simulink library "SV_pattern_generator_with_global_TRGO"  (R2025b)
settings: Solver=VariableStepAuto  StartTime=0.0  StopTime=10.0  RelTol=1e-3
undefined symbols (not defined in the file): fPWM_DAB, tc
libraries: single_phase_pwm_modulator x1
settings Model: Creator=dbagn  LastModifiedBy=dbagn

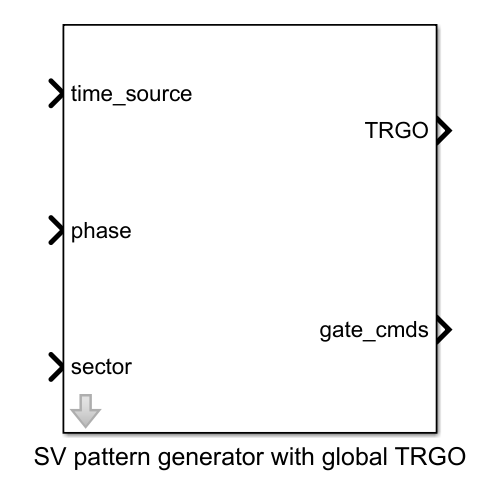
[thumbnail: Simulink's stored preview of the top-level diagram]
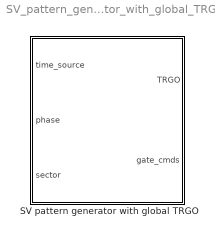
== system SV_pattern_generator_with_global_TRGO ==
  SV pattern generator with global TRGO : Subsystem  mask{f=fPWM_DAB, m_up=0.98, m_low=0.02, dead_time=0, pos_cmd_gate=15, neg_cmd_gate=-10, tc=tc}
      mask prompts: f "Frequency (Hz)"; m_up "Max Input Modulation Value"; m_low "Min Input Modulation Value"; dead_time "Dead Time (s)"; pos_cmd_gate "Positive Gate Voltage (V)"; neg_cmd_gate "Negative Gate Voltage (V)"; tc "Sampling time (s)"

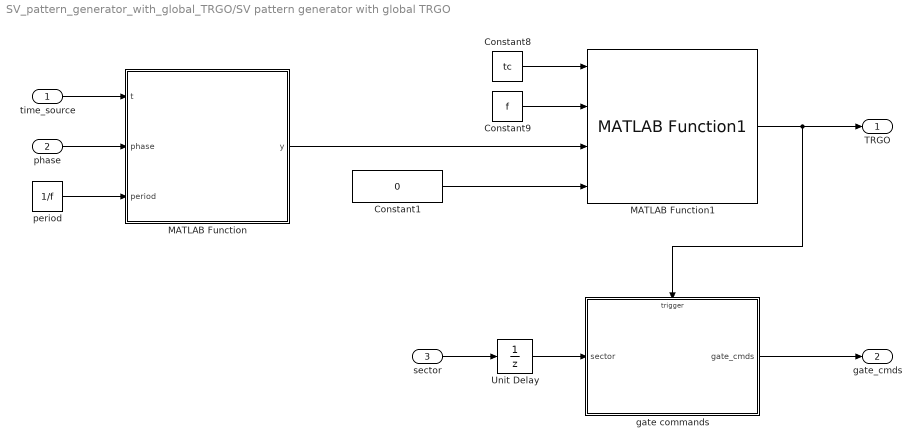
== system SV_pattern_generator_with_global_TRGO/SV pattern generator with global TRGO ==
  time_source : Inport
  phase : Inport  Port=2
  sector : Inport  Port=3
  Constant1 : Constant  Value=0
  Constant8 : Constant  Value=tc
  Constant9 : Constant  Value=f
  MATLAB Function : MATLAB Function  TreatAsAtomicUnit=on  SystemSampleTime=tc
  MATLAB Function1 : single_phase_pwm_modulator/Single phase two level PWM generator with global TRGO/MATLAB Function1  SystemSampleTime=tc  VariantActivationTime=update diagram  EmptyChoice=off  PassThrough=off  PassThroughVariantControl=(default)  EmptyChoiceVariantControl=(default)  AllowFlexibleInterface=on  Latency=0  AutoFrameSizeCalculation=off
  Unit Delay : UnitDelay  SampleTime=tc  HasFrameUpgradeWarning=on
  gate commands : Subsystem
  period : Constant  Value=1/f
  TRGO : Outport
  gate_cmds : Outport  Port=2
  wires:
  Constant1/1 -> MATLAB Function1/4
  time_source/1 -> MATLAB Function/1(t)
  gate commands/1(gate_cmds) -> gate_cmds/1
  sector/1 -> Unit Delay/1
  Constant9/1 -> MATLAB Function1/2
  Constant8/1 -> MATLAB Function1/1
  MATLAB Function/1(y) -> MATLAB Function1/3
  phase/1 -> MATLAB Function/2(phase)
  period/1 -> MATLAB Function/3(period)
  MATLAB Function1/1 -> gate commands/Trigger, TRGO/1
  Unit Delay/1 -> gate commands/1(sector)

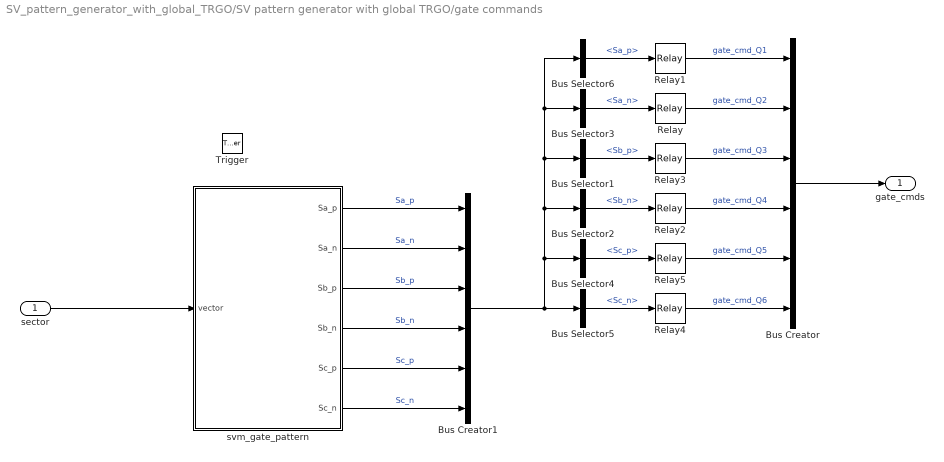
== system SV_pattern_generator_with_global_TRGO/SV pattern generator with global TRGO/gate commands ==
  sector : Inport
  Trigger : TriggerPort  VariantControl=(inherit)  PortDimensions=1
  Bus Creator : BusCreator  Inputs=6
  Bus Creator1 : BusCreator  Inputs=6
  Bus Selector1 : BusSelector  OutputSignals=Sb_p
  Bus Selector2 : BusSelector  OutputSignals=Sb_n
  Bus Selector3 : BusSelector  OutputSignals=Sa_n
  Bus Selector4 : BusSelector  OutputSignals=Sc_p
  Bus Selector5 : BusSelector  OutputSignals=Sc_n
  Bus Selector6 : BusSelector  OutputSignals=Sa_p
  Relay{,1..5} (6 alike) : Relay  OnOutputValue=pos_cmd_gate  OffOutputValue=neg_cmd_gate
  svm_gate_pattern : MATLAB Function  TreatAsAtomicUnit=on
  gate_cmds : Outport
  wires:
  Bus Selector2/1 -> Relay2/1  "<Sb_n>"
  Relay5/1 -> Bus Creator/5  "gate_cmd_Q5"
  Relay1/1 -> Bus Creator/1  "gate_cmd_Q1"
  Relay/1 -> Bus Creator/2  "gate_cmd_Q2"
  Bus Selector1/1 -> Relay3/1  "<Sb_p>"
  Relay3/1 -> Bus Creator/3  "gate_cmd_Q3"
  Bus Selector6/1 -> Relay1/1  "<Sa_p>"
  Bus Selector4/1 -> Relay5/1  "<Sc_p>"
  Bus Selector5/1 -> Relay4/1  "<Sc_n>"
  Relay2/1 -> Bus Creator/4  "gate_cmd_Q4"
  Bus Selector3/1 -> Relay/1  "<Sa_n>"
  Bus Creator/1 -> gate_cmds/1
  Relay4/1 -> Bus Creator/6  "gate_cmd_Q6"
  sector/1 -> svm_gate_pattern/1(vector)
  svm_gate_pattern/1(Sa_p) -> Bus Creator1/1  "Sa_p"
  svm_gate_pattern/2(Sa_n) -> Bus Creator1/2  "Sa_n"
  svm_gate_pattern/3(Sb_p) -> Bus Creator1/3  "Sb_p"
  svm_gate_pattern/4(Sb_n) -> Bus Creator1/4  "Sb_n"
  svm_gate_pattern/5(Sc_p) -> Bus Creator1/5  "Sc_p"
  svm_gate_pattern/6(Sc_n) -> Bus Creator1/6  "Sc_n"
  Bus Creator1/1 -> Bus Selector4/1, Bus Selector2/1, Bus Selector1/1, Bus Selector3/1, Bus Selector6/1, Bus Selector5/1

== matlab function SV_pattern_generator_with_global_TRGO/SV pattern generator with global TRGO/gate commands/svm_gate_pattern ==
  data: vector input; Sa_p output; Sa_n output; Sb_p output; Sb_n output; Sc_p output; Sc_n output
function [Sa_p,Sa_n,Sb_p,Sb_n,Sc_p,Sc_n] = svm_gate_pattern(vector)

% upper = [Sa+ Sb+ Sc+]
% lower = [Sa− Sb− Sc−]
switch vector
    case 0
        % u0 [Sa+ Sb+ Sc+] = [0 0 0]
        upper = [0 0 0];
    case 1
        % u1 [Sa+ Sb+ Sc+] = [1 0 0]
        upper = [1 0 0];
    case 2
        % u2 [Sa+ Sb+ Sc+] = [1 1 0]
        upper = [1 1 0];
    case 3
        % u3 [Sa+ Sb+ Sc+] = [0 1 0]
        upper = [0 1 0];
    case 4
        % u4 [Sa+ Sb+ Sc+] = [0 1 1]
        upper = [0 1 1];
    case 5
        % u5 [Sa+ Sb+ Sc+] = [0 0 1]
        upper = [0 0 1];
    case 6
        % u6 [Sa+ Sb+ Sc+] = [1 0 1]
        upper = [1 0 1];
    case 7
        % u7 = u0 [Sa+ Sb+ Sc+] = [1 1 1]
        upper = [1 1 1];
    otherwise
        % otherwise
        upper = [0 0 0];
end

lower = 1 - upper;

Sa_p = upper(1);
Sb_p = upper(2);
Sc_p = upper(3);
Sa_n = lower(1);
Sb_n = lower(2);
Sc_n = lower(3);

% output [Sa+ Sa− Sb+ Sb− Sc+  Sc−]

end

== matlab function SV_pattern_generator_with_global_TRGO/SV pattern generator with global TRGO/MATLAB Function ==
  data: t input; y output; phase input; period input
function y = ramp_up_down(t,phase,period)
x = sin(2*pi/period*t - phase -pi/2);
y = asin(x)/pi + 1/2;
